simulink model "Lab6_jinjin"  (R2022a)
settings: Solver=VariableStepAuto  StartTime=0.0  StopTime=1200  RelTol=1e-3
libraries: matrix_library x4, sharedutil x2
settings Model: Creator=Administrator  LastModifiedBy=이진진
settings DebuggingCC: UnconnectedInputMsg=warning  UnconnectedOutputMsg=warning  UnconnectedLineMsg=warning
settings RTWCC: DLArmComputeVersion=19.05

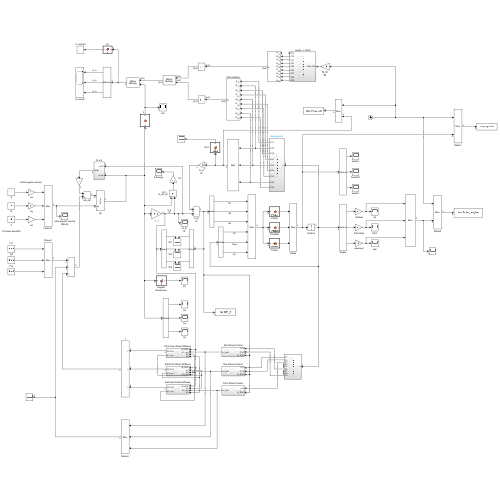
[thumbnail: Simulink's stored preview of the top-level diagram]
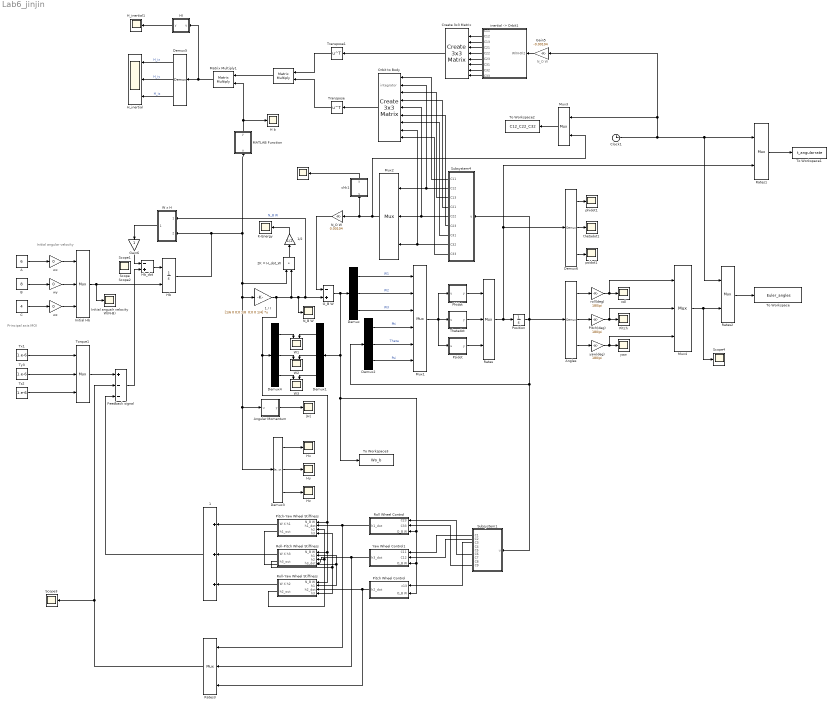
== system Lab6_jinjin ==
  note: Initial angular velocity
  note: Principal axis MOI
  note: N_O
      | W
  note: integrator
  " " : Scope
  "  " : Product  Multiplication=Matrix(*)
  " 1" : Sum  Inputs=+++
  1 / I : Gain  Gain="[1/6 0 0;0 1/8  0;0 0 1/4]"  Multiplication=Matrix(K*u)
  1/2 : Gain  Gain=1/2
  2K = H_dot_W : DotProduct  OutDataTypeStr=Inherit: Inherit via internal rule
  A : Constant  Value=6
  Angles : Demux  Outputs=3
      settings: DisplayOption=none
  Angular Momentum : MATLAB Function  TreatAsAtomicUnit=on
  B : Constant  Value=8
  C : Constant  Value=4
  Clock1 : Clock
  Create 3x3 Matrix : sharedutil/Create 3x3 Matrix  aMode=aMode
      settings: SourceProductBaseCode=AE,PW,DR,MT,VE
  Demux{,1..6} (7 alike) : Demux  Outputs=3
      settings: DisplayOption=none
  Feedback signal : Sum  Inputs=+--
  Gain5 : Gain  Gain=-0.00104
  Gain6 : Gain
  H b : Scope
  HI : MATLAB Function  TreatAsAtomicUnit=on
  H_inertial : Scope  NumInputPorts=3
  H_inertial1 : Scope
  Hb : Integrator  InitialConditionSource=external  InitialCondition=[0.2;0.3;0.4]
  Hb_dot : Sum  Inputs=-+
  Hx : Scope
  Hy : Scope
  Hz : Scope
  Initial Hb : Mux  Inputs=3
  Initial angualr velocity W(N-B) : Scope
  K-Energy : Scope
  MATLAB Function : MATLAB Function  TreatAsAtomicUnit=on
  Matrix Multiply1 : Product  Multiplication=Matrix(*)
  Mux1 : Mux  Inputs=6
  Mux2 : Mux  Inputs=3
  Mux3 : Mux  Inputs=2
  Mux4 : Mux  Inputs=3
  N_B W : Scope
  N_O W : Gain  Gain=0.00104
  O_B W : Sum  Inputs=-+
  Orbit to Body : sharedutil/Create 3x3 Matrix  aMode=aMode
      settings: SourceProductBaseCode=AE,PW,DR,MT,VE
  Phidot : MATLAB Function  TreatAsAtomicUnit=on
  Pitch : Scope
  Pitch Wheel Control : Subsystem
  Pitch(deg) : Gain  Gain=180/pi
  Pitch-Yaw Wheel Stiffness : Subsystem
  Position : Integrator  InitialCondition=[5*pi/180 5*pi/180 5*pi/180]
  Psidot : MATLAB Function  TreatAsAtomicUnit=on
  Rates : Mux  Inputs=3
  Rates1 : Mux  Inputs=2
  Rates2 : Mux  Inputs=2
  Rates3 : Mux  Inputs=3
  Roll Wheel Control : Subsystem
  Roll-Pitch Wheel Stiffness : Subsystem
  Roll-Yaw Wheel Stiffness : Subsystem
  Scope{,1..4} (5 alike) : Scope
  Subsystem1 : Subsystem
  Subsystem4 : Subsystem
  Thetadot : MATLAB Function  TreatAsAtomicUnit=on
  To Workspace : ToWorkspace  VariableName=Euler_angles  SampleTime=-1
  To Workspace1 : ToWorkspace  VariableName=t_angularrate  SaveFormat=Timeseries  SampleTime=-1
  To Workspace2 : ToWorkspace  VariableName=C12_C22_C32  SaveFormat=Timeseries  SampleTime=-1
  To Workspace3 : ToWorkspace  VariableName=Wo_b  SaveFormat=Timeseries  SampleTime=-1
  Torque1 : Mux  Inputs=3
  Transpose : Math  Operator=transpose
  Transpose1 : Math  Operator=transpose
  Tx1 : Constant  Value=1.e-6
  Ty3 : Constant  Value=1.e-6
  Tz2 : Constant  Value=1.e-6
  W x H : Subsystem
  W1 : Scope  NumInputPorts=2
  W2 : Scope  NumInputPorts=2
  W3 : Scope  NumInputPorts=2
  Yaw Wheel Control1 : Subsystem
  chk1 : MATLAB Function  TreatAsAtomicUnit=on
  "inertial -> Orbit1" : Subsystem
  phidot1 : Scope
  psidot1 : Scope
  roll : Scope
  roll(deg) : Gain  Gain=180/pi
  thetadot1 : Scope
  wx : Gain  Gain=0
  wy : Gain  Gain=0
  wz : Gain  Gain=0
  yaw : Scope
  yaw(deg) : Gain  Gain=180/pi
  |H| : Scope
  wires:
  Hb_dot/1 -> Hb/1
  W x H/1(WxH) -> Gain6/1
  Thetadot/1(y) -> Rates/2
  Demux2/1 -> Mux1/4  "Phi"
  Phidot/1(y) -> Rates/1
  Demux2/3 -> Mux1/6  "Psi"
  Demux1/2 -> W2/2
  Demux/3 -> Mux1/3  "W3"
  O_B W/1 -> Demux1/1, To Workspace3/1, Pitch Wheel Control/2(O_B W), Yaw Wheel Control1/3(O_B W), Roll Wheel Control/3(O_B W), Demux/1
  Subsystem4/2(C12) -> Mux2/1, Orbit to Body/2
  roll(deg)/1 -> Mux4/1, roll/1
  Angles/2 -> Pitch(deg)/1
  yaw(deg)/1 -> Mux4/3, yaw/1
  Angles/1 -> roll(deg)/1
  Demux/2 -> Mux1/2  "W2"
  "  "/1 -> Matrix Multiply1/1
  Subsystem4/1(C11) -> Orbit to Body/1
  Transpose/1 -> "  "/2
  Subsystem4/4(C21) -> Orbit to Body/4
  1 / I/1 -> Roll-Pitch Wheel Stiffness/1(N_B W), Roll-Yaw Wheel Stiffness/1(N_B W), Pitch-Yaw Wheel Stiffness/1(N_B W), Demux4/1, N_B W/1, W x H/1(in W), O_B W/2, 2K = H_dot_W/2  "N_B W"
  Transpose1/1 -> "  "/1
  Orbit to Body/1 -> Transpose/1
  Create 3x3 Matrix/1 -> Transpose1/1
  Demux1/3 -> W3/2
  Subsystem4/9(C33) -> Orbit to Body/9
  Angles/3 -> yaw(deg)/1
  2K = H_dot_W/1 -> 1/2/1
  chk1/1(y) -> " "/1
  Demux3/3 -> Hz/1
  Gain5/1 -> "inertial -> Orbit1"/1(W(N-O)2)
  Demux3/2 -> Hy/1
  Psidot/1(y) -> Rates/3
  Mux4/1 -> Scope4/1, Rates2/2
  Demux6/1 -> phidot1/1
  Demux6/2 -> thetadot1/1
  Subsystem4/6(C23) -> Orbit to Body/6
  Mux2/1 -> Mux3/2, chk1/1(u), N_O W/1
  Demux3/1 -> Hx/1
  Subsystem4/5(C22) -> Orbit to Body/5, Mux2/2
  N_O W/1 -> O_B W/1
  Demux/1 -> Mux1/1  "W1"
  Angular Momentum/1(y) -> |H|/1
  Demux2/2 -> Mux1/5  "Theta"
  Subsystem4/7(C31) -> Orbit to Body/7
  Hb/1 -> W x H/2(in Hb), Angular Momentum/1(u), Demux3/1, 1 / I/1, 2K = H_dot_W/1, MATLAB Function/1(u)
  Demux6/3 -> psidot1/1
  MATLAB Function/1(y) -> H b/1, Matrix Multiply1/2
  Mux1/1 -> Thetadot/1(u), Psidot/1(u), Phidot/1(u)
  Subsystem4/8(C32) -> Orbit to Body/8, Mux2/3
  Subsystem4/3(C13) -> Orbit to Body/3
  1/2/1 -> K-Energy/1
  C/1 -> wz/1
  B/1 -> wy/1
  Initial Hb/1 -> Hb/2, Initial angualr velocity W(N-B)/1
  wy/1 -> Initial Hb/2
  Ty3/1 -> Torque1/2
  wz/1 -> Initial Hb/3
  A/1 -> wx/1
  Torque1/1 -> Feedback signal/1
  Tz2/1 -> Torque1/3
  wx/1 -> Initial Hb/1
  Tx1/1 -> Torque1/1
  Feedback signal/1 -> Hb_dot/2
  Demux5/2 -> H_inertial/2  "H_iy"
  HI/1(y) -> H_inertial1/1
  Demux5/1 -> H_inertial/1  "H_ix"
  Matrix Multiply1/1 -> HI/1(u), Demux5/1
  Demux5/3 -> H_inertial/3  "H_iz"
  Position/1 -> Subsystem4/1(u), Subsystem1/1(u), Demux2/1, Angles/1
  Gain6/1 -> Hb_dot/1
  Rates1/1 -> To Workspace1/1
  Rates2/1 -> To Workspace/1
  Rates/1 -> Position/1, Rates1/2, Demux6/1
  Mux3/1 -> To Workspace2/1
  Clock1/1 -> Gain5/1, Mux3/1, Rates1/1, Rates2/1
  Subsystem1/3(C3) -> Pitch Wheel Control/1(c13)
  Subsystem1/1(C1) -> Yaw Wheel Control1/1(C11)
  Subsystem1/2(C2) -> Yaw Wheel Control1/2(C12)
  Subsystem1/6(C6) -> Roll Wheel Control/1(C23)
  Subsystem1/9(C9) -> Roll Wheel Control/2(C33)
  Roll Wheel Control/1(h1_dot) -> Rates3/1, Pitch-Yaw Wheel Stiffness/2(h1_dot)
  Pitch Wheel Control/1(h2_dot) -> Rates3/3, Roll-Yaw Wheel Stiffness/3(h2_dot)
  Yaw Wheel Control1/1(h3_dot) -> Rates3/2, Roll-Pitch Wheel Stiffness/4(h3_dot)
  Roll-Yaw Wheel Stiffness/2(h2_out) -> Pitch-Yaw Wheel Stiffness/3(h2), Roll-Pitch Wheel Stiffness/3(h2)
  Roll-Pitch Wheel Stiffness/2(h3_out) -> Roll-Yaw Wheel Stiffness/4(h3), Pitch-Yaw Wheel Stiffness/4(h3)
  Pitch-Yaw Wheel Stiffness/2(h1_out) -> Roll-Yaw Wheel Stiffness/2(h1), Roll-Pitch Wheel Stiffness/2(h1)
  Pitch-Yaw Wheel Stiffness/1(W X h1) -> " 1"/1
  Roll-Yaw Wheel Stiffness/1(W X h2) -> " 1"/3
  Roll-Pitch Wheel Stiffness/1(W X h3) -> " 1"/2
  " 1"/1 -> Feedback signal/3
  Rates3/1 -> Feedback signal/2, Scope3/1
  Demux1/1 -> W1/2
  Demux4/1 -> W1/1
  Demux4/2 -> W2/1
  Demux4/3 -> W3/1
  Pitch(deg)/1 -> Mux4/2, Pitch/1
  "inertial -> Orbit1"/9("C33 ") -> Create 3x3 Matrix/9
  "inertial -> Orbit1"/8("C32 ") -> Create 3x3 Matrix/8
  "inertial -> Orbit1"/5("C22 ") -> Create 3x3 Matrix/5
  "inertial -> Orbit1"/7("C31 ") -> Create 3x3 Matrix/7
  "inertial -> Orbit1"/6("C23 ") -> Create 3x3 Matrix/6
  "inertial -> Orbit1"/2("C12 ") -> Create 3x3 Matrix/2
  "inertial -> Orbit1"/3("C13 ") -> Create 3x3 Matrix/3
  "inertial -> Orbit1"/4("C21 ") -> Create 3x3 Matrix/4

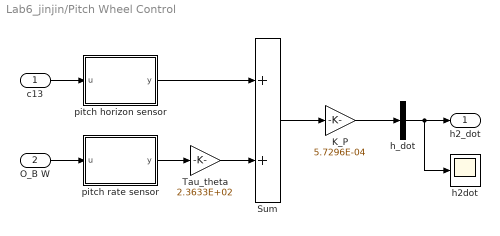
== system Lab6_jinjin/Pitch Wheel Control ==
  c13 : Inport
  O_B W : Inport  Port=2
  K_P : Gain  Gain=5.7296E-04
  Sum : Sum
  Tau_theta : Gain  Gain=2.3633E+02
  h2dot : Scope
  h_dot : Mux  Inputs=1
  pitch horizon sensor : MATLAB Function  TreatAsAtomicUnit=on
  pitch rate sensor : MATLAB Function  TreatAsAtomicUnit=on
  h2_dot : Outport
  wires:
  K_P/1 -> h_dot/1
  h_dot/1 -> h2dot/1, h2_dot/1
  pitch horizon sensor/1(y) -> Sum/1
  Tau_theta/1 -> Sum/2
  pitch rate sensor/1(y) -> Tau_theta/1
  O_B W/1 -> pitch rate sensor/1(u)
  c13/1 -> pitch horizon sensor/1(u)
  Sum/1 -> K_P/1

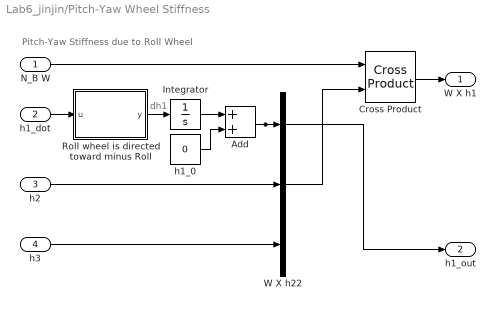
== system Lab6_jinjin/Pitch-Yaw Wheel Stiffness ==
  note: Pitch-Yaw Stiffness due to Roll Wheel
  note: dh1
  N_B W : Inport
  h1_dot : Inport  Port=2
  h2 : Inport  Port=3
  h3 : Inport  Port=4
  Add : Sum
  Cross Product : matrix_library/Cross Product
      settings: SourceProductBaseCode=SL
  Integrator : Integrator  InitialCondition=.0
  Roll wheel is directed toward minus Roll : MATLAB Function  TreatAsAtomicUnit=on
  W X h22 : Mux  Inputs=3
  h1_0 : Constant  Value=0  VectorParams1D=off
  W X h1 : Outport
  h1_out : Outport  Port=2
  wires:
  h1_dot/1 -> Roll wheel is directed toward minus Roll/1(u)
  Roll wheel is directed toward minus Roll/1(y) -> Integrator/1
  h1_0/1 -> Add/2
  Integrator/1 -> Add/1
  h3/1 -> W X h22/3
  N_B W/1 -> Cross Product/1
  W X h22/1 -> Cross Product/2
  Cross Product/1 -> W X h1/1
  h2/1 -> W X h22/2
  Add/1 -> h1_out/1, W X h22/1

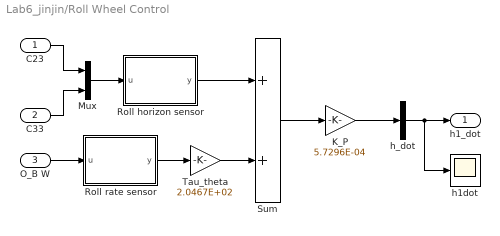
== system Lab6_jinjin/Roll Wheel Control ==
  C23 : Inport
  C33 : Inport  Port=2
  O_B W : Inport  Port=3
  K_P : Gain  Gain=5.7296E-04
  Mux : Mux  Inputs=2
  Roll horizon sensor : MATLAB Function  TreatAsAtomicUnit=on
  Roll rate sensor : MATLAB Function  TreatAsAtomicUnit=on
  Sum : Sum
  Tau_theta : Gain  Gain=2.0467E+02
  h1dot : Scope
  h_dot : Mux  Inputs=1
  h1_dot : Outport
  wires:
  K_P/1 -> h_dot/1
  h_dot/1 -> h1dot/1, h1_dot/1
  Roll horizon sensor/1(y) -> Sum/1
  Tau_theta/1 -> Sum/2
  Roll rate sensor/1(y) -> Tau_theta/1
  O_B W/1 -> Roll rate sensor/1(u)
  Sum/1 -> K_P/1
  C23/1 -> Mux/1
  C33/1 -> Mux/2
  Mux/1 -> Roll horizon sensor/1(u)

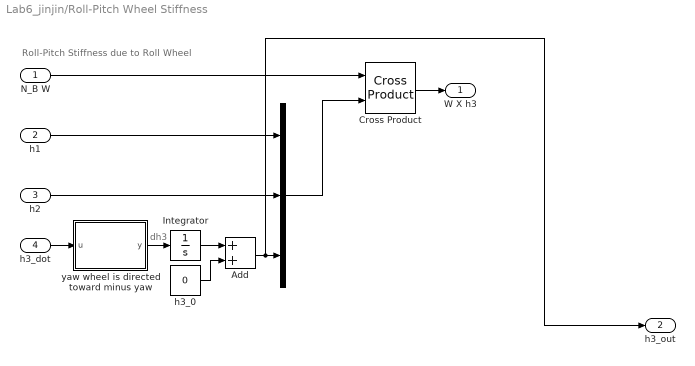
== system Lab6_jinjin/Roll-Pitch Wheel Stiffness ==
  note: Roll-Pitch Stiffness due to Roll Wheel
  note: dh3
  N_B W : Inport
  h1 : Inport  Port=2
  h2 : Inport  Port=3
  h3_dot : Inport  Port=4
  " " : Mux  Inputs=3
  Add : Sum
  Cross Product : matrix_library/Cross Product
      settings: SourceProductBaseCode=SL
  Integrator : Integrator  InitialCondition=.0
  h3_0 : Constant  Value=0  VectorParams1D=off
  yaw wheel is directed toward minus yaw : MATLAB Function  TreatAsAtomicUnit=on
  W X h3 : Outport
  h3_out : Outport  Port=2
  wires:
  h3_dot/1 -> yaw wheel is directed toward minus yaw/1(u)
  yaw wheel is directed toward minus yaw/1(y) -> Integrator/1
  h3_0/1 -> Add/2
  Integrator/1 -> Add/1
  N_B W/1 -> Cross Product/1
  " "/1 -> Cross Product/2
  Cross Product/1 -> W X h3/1
  Add/1 -> h3_out/1, " "/3
  h1/1 -> " "/1
  h2/1 -> " "/2

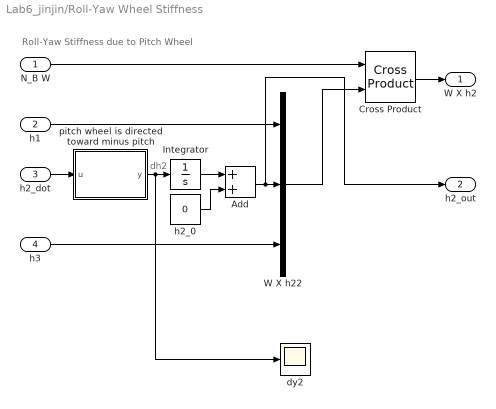
== system Lab6_jinjin/Roll-Yaw Wheel Stiffness ==
  note: Roll-Yaw Stiffness due to Pitch Wheel
  note: dh2
  N_B W : Inport
  h1 : Inport  Port=2
  h2_dot : Inport  Port=3
  h3 : Inport  Port=4
  Add : Sum
  Cross Product : matrix_library/Cross Product
      settings: SourceProductBaseCode=SL
  Integrator : Integrator  InitialCondition=.0
  W X h22 : Mux  Inputs=3
  dy2 : Scope
  h2_0 : Constant  Value=0  VectorParams1D=off
  pitch wheel is directed toward minus pitch : MATLAB Function  TreatAsAtomicUnit=on
  W X h2 : Outport
  h2_out : Outport  Port=2
  wires:
  h2_dot/1 -> pitch wheel is directed toward minus pitch/1(u)
  pitch wheel is directed toward minus pitch/1(y) -> dy2/1, Integrator/1
  Add/1 -> h2_out/1, W X h22/2
  h2_0/1 -> Add/2
  Integrator/1 -> Add/1
  h3/1 -> W X h22/3
  h1/1 -> W X h22/1
  N_B W/1 -> Cross Product/1
  W X h22/1 -> Cross Product/2
  Cross Product/1 -> W X h2/1

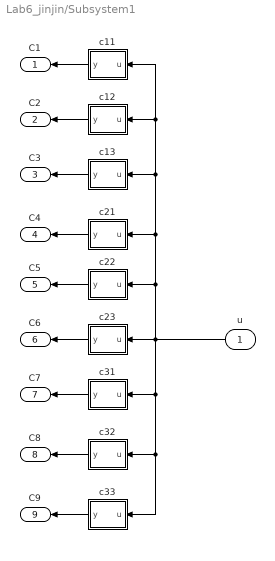
== system Lab6_jinjin/Subsystem1 ==
  u : Inport
  c11 : MATLAB Function  TreatAsAtomicUnit=on
  c12 : MATLAB Function  TreatAsAtomicUnit=on
  c13 : MATLAB Function  TreatAsAtomicUnit=on
  c21 : MATLAB Function  TreatAsAtomicUnit=on
  c22 : MATLAB Function  TreatAsAtomicUnit=on
  c23 : MATLAB Function  TreatAsAtomicUnit=on
  c31 : MATLAB Function  TreatAsAtomicUnit=on
  c32 : MATLAB Function  TreatAsAtomicUnit=on
  c33 : MATLAB Function  TreatAsAtomicUnit=on
  C1 : Outport
  C2 : Outport  Port=2
  C3 : Outport  Port=3
  C4 : Outport  Port=4
  C5 : Outport  Port=5
  C6 : Outport  Port=6
  C7 : Outport  Port=7
  C8 : Outport  Port=8
  C9 : Outport  Port=9
  wires:
  c32/1(y) -> C8/1
  c33/1(y) -> C9/1
  c23/1(y) -> C6/1
  c22/1(y) -> C5/1
  c12/1(y) -> C2/1
  c31/1(y) -> C7/1
  c13/1(y) -> C3/1
  c21/1(y) -> C4/1
  u/1 -> c32/1(u), c33/1(u), c31/1(u), c22/1(u), c13/1(u), c12/1(u), c11/1(u), c21/1(u), c23/1(u)
  c11/1(y) -> C1/1

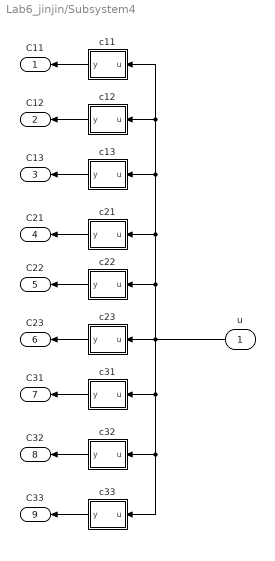
== system Lab6_jinjin/Subsystem4 ==
  u : Inport
  c11 : MATLAB Function  TreatAsAtomicUnit=on
  c12 : MATLAB Function  TreatAsAtomicUnit=on
  c13 : MATLAB Function  TreatAsAtomicUnit=on
  c21 : MATLAB Function  TreatAsAtomicUnit=on
  c22 : MATLAB Function  TreatAsAtomicUnit=on
  c23 : MATLAB Function  TreatAsAtomicUnit=on
  c31 : MATLAB Function  TreatAsAtomicUnit=on
  c32 : MATLAB Function  TreatAsAtomicUnit=on
  c33 : MATLAB Function  TreatAsAtomicUnit=on
  C11 : Outport
  C12 : Outport  Port=2
  C13 : Outport  Port=3
  C21 : Outport  Port=4
  C22 : Outport  Port=5
  C23 : Outport  Port=6
  C31 : Outport  Port=7
  C32 : Outport  Port=8
  C33 : Outport  Port=9
  wires:
  c22/1(y) -> C22/1
  c21/1(y) -> C21/1
  c23/1(y) -> C23/1
  c33/1(y) -> C33/1
  c32/1(y) -> C32/1
  c12/1(y) -> C12/1
  c11/1(y) -> C11/1
  u/1 -> c32/1(u), c33/1(u), c31/1(u), c22/1(u), c13/1(u), c12/1(u), c11/1(u), c21/1(u), c23/1(u)
  c31/1(y) -> C31/1
  c13/1(y) -> C13/1

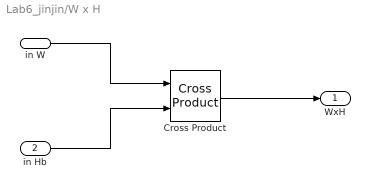
== system Lab6_jinjin/W x H ==
  in W : Inport
  in Hb : Inport  Port=2
  Cross Product : matrix_library/Cross Product
      settings: SourceProductBaseCode=SL
  WxH : Outport
  wires:
  in W/1 -> Cross Product/1
  Cross Product/1 -> WxH/1
  in Hb/1 -> Cross Product/2

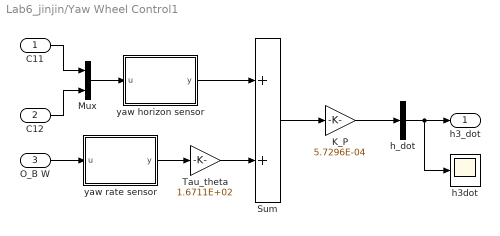
== system Lab6_jinjin/Yaw Wheel Control1 ==
  C11 : Inport
  C12 : Inport  Port=2
  O_B W : Inport  Port=3
  K_P : Gain  Gain=5.7296E-04
  Mux : Mux  Inputs=2
  Sum : Sum
  Tau_theta : Gain  Gain=1.6711E+02
  h3dot : Scope
  h_dot : Mux  Inputs=1
  yaw horizon sensor : MATLAB Function  TreatAsAtomicUnit=on
  yaw rate sensor : MATLAB Function  TreatAsAtomicUnit=on
  h3_dot : Outport
  wires:
  K_P/1 -> h_dot/1
  h_dot/1 -> h3dot/1, h3_dot/1
  yaw horizon sensor/1(y) -> Sum/1
  Tau_theta/1 -> Sum/2
  yaw rate sensor/1(y) -> Tau_theta/1
  O_B W/1 -> yaw rate sensor/1(u)
  Sum/1 -> K_P/1
  Mux/1 -> yaw horizon sensor/1(u)
  C11/1 -> Mux/1
  C12/1 -> Mux/2

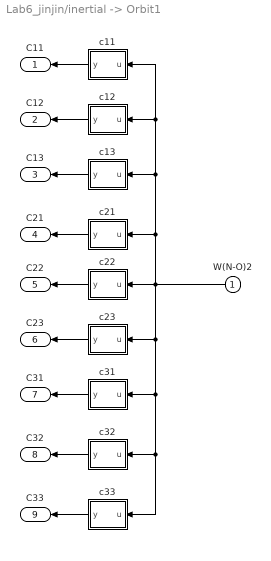
== system Lab6_jinjin/inertial -> Orbit1 ==
  W(N-O)2 : Inport
  c11 : MATLAB Function  TreatAsAtomicUnit=on
  c12 : MATLAB Function  TreatAsAtomicUnit=on
  c13 : MATLAB Function  TreatAsAtomicUnit=on
  c21 : MATLAB Function  TreatAsAtomicUnit=on
  c22 : MATLAB Function  TreatAsAtomicUnit=on
  c23 : MATLAB Function  TreatAsAtomicUnit=on
  c31 : MATLAB Function  TreatAsAtomicUnit=on
  c32 : MATLAB Function  TreatAsAtomicUnit=on
  c33 : MATLAB Function  TreatAsAtomicUnit=on
  "C11 " : Outport
  "C12 " : Outport  Port=2
  "C13 " : Outport  Port=3
  "C21 " : Outport  Port=4
  "C22 " : Outport  Port=5
  "C23 " : Outport  Port=6
  "C31 " : Outport  Port=7
  "C32 " : Outport  Port=8
  "C33 " : Outport  Port=9
  wires:
  c13/1(y) -> "C13 "/1
  c33/1(y) -> "C33 "/1
  c21/1(y) -> "C21 "/1
  c22/1(y) -> "C22 "/1
  c11/1(y) -> "C11 "/1
  c12/1(y) -> "C12 "/1
  W(N-O)2/1 -> c13/1(u), c12/1(u), c11/1(u), c21/1(u), c32/1(u), c33/1(u), c31/1(u), c23/1(u), c22/1(u)
  c32/1(y) -> "C32 "/1
  c31/1(y) -> "C31 "/1
  c23/1(y) -> "C23 "/1

== matlab function Lab6_jinjin/Angular Momentum ==
  data: u input; y output
function y = f(u)

y = sqrt(u(1)^2 + u(2)^2 + u(3)^2);

end

== matlab function Lab6_jinjin/Subsystem1/c12 ==
  data: u input; y output
function y = fcn(u)

y = sin(u(3))*cos(u(2));

== matlab function Lab6_jinjin/Subsystem1/c13 ==
  data: u input; y output
function y = fcn(u)

y = -sin(u(2));

== matlab function Lab6_jinjin/chk1 ==
  data: u input; y output
function y = chk1(u)

y = u(1)^2+u(2)^2+u(3)^2-1

end

== matlab function Lab6_jinjin/Subsystem4/c32 ==
  data: u input; y output
function y = fcn(u)

y = -cos(u(3))*sin(u(1))+sin(u(3))*sin(u(2))*cos(u(1));

== matlab function Lab6_jinjin/inertial -> Orbit1/c12 ==
  data: u input; y output
function y = fcn(u)

y = 0;

== matlab function Lab6_jinjin/Subsystem4/c33 ==
  data: u input; y output
function y = fcn(u)

y = cos(u(2))*cos(u(1));

== matlab function Lab6_jinjin/Subsystem1/c21 ==
  data: u input; y output
function y = fcn(u)

y = -sin(u(3))*cos(u(1))+cos(u(3))*sin(u(2))*sin(u(1));

== matlab function Lab6_jinjin/Subsystem1/c22 ==
  data: u input; y output
function y = fcn(u)

y = cos(u(3))*cos(u(1))+sin(u(3))*sin(u(2))*sin(u(1));

== matlab function Lab6_jinjin/Subsystem1/c23 ==
  data: u input; y output
function y = fcn(u)

y = cos(u(2))*sin(u(1));

== matlab function Lab6_jinjin/Subsystem1/c31 ==
  data: u input; y output
function y = fcn(u)

y = sin(u(3))*sin(u(1))+cos(u(3))*sin(u(2))*cos(u(1));

== matlab function Lab6_jinjin/Subsystem1/c32 ==
  data: u input; y output
function y = fcn(u)

y = -cos(u(3))*sin(u(1))+sin(u(3))*sin(u(2))*cos(u(1));

== matlab function Lab6_jinjin/Subsystem1/c33 ==
  data: u input; y output
function y = fcn(u)

y = cos(u(2))*cos(u(1));

== matlab function Lab6_jinjin/Pitch Wheel Control/pitch horizon sensor ==
  data: u input; y output
function y = fcn(u)

y = -u(1);

== matlab function Lab6_jinjin/MATLAB Function ==
  data: u input; y output
function y = f(u)

y = zeros(3,1);

y(1,1) = u(1);
y(2,1) = u(2);
y(3,1) = u(3);

== matlab function Lab6_jinjin/Pitch Wheel Control/pitch rate sensor ==
  data: u input; y output
function y = fcn(u)

y = u(2);

== matlab function Lab6_jinjin/inertial -> Orbit1/c13 ==
  data: u input; y output
function y = fcn(u)

y = -sin(u);

== matlab function Lab6_jinjin/Roll Wheel Control/Roll horizon sensor ==
  data: u input; y output
function y = fcn(u)

y = atan(u(1)/u(2));

== matlab function Lab6_jinjin/HI ==
  data: u input; y output
function y = fcn(u)

y = sqrt((u(1)^2+u(2)^2+u(3)^2));

== matlab function Lab6_jinjin/Roll Wheel Control/Roll rate sensor ==
  data: u input; y output
function y = fcn(u)

y = u(1);

== matlab function Lab6_jinjin/Yaw Wheel Control1/yaw horizon sensor ==
  data: u input; y output
function y = fcn(u)

y = atan(u(2)/u(1));

== matlab function Lab6_jinjin/Yaw Wheel Control1/yaw rate sensor ==
  data: u input; y output
function y = fcn(u)

y = u(3);

== matlab function Lab6_jinjin/Pitch-Yaw Wheel Stiffness/Roll wheel is directed toward minus Roll ==
  data: u input; y output
function y = fcn(u)

y = -u(1);

== matlab function Lab6_jinjin/Roll-Pitch Wheel Stiffness/yaw wheel is directed toward minus yaw ==
  data: u input; y output
function y = fcn(u)

y = -u(1);

== matlab function Lab6_jinjin/Roll-Yaw Wheel Stiffness/pitch wheel is directed toward minus pitch ==
  data: u input; y output
function y = fcn(u)

y = -u(1);

== matlab function Lab6_jinjin/inertial -> Orbit1/c21 ==
  data: u input; y output
function y = fcn(u)

y = 0;

== matlab function Lab6_jinjin/inertial -> Orbit1/c22 ==
  data: u input; y output
function y = fcn(u)

y = 1;

== matlab function Lab6_jinjin/Phidot ==
  data: u input; y output
function y = Phidot(u)

y = u(1) + sin(u(4))*tan(u(5))*u(2) + cos(u(4))*tan(u(5))*u(3);

end

== matlab function Lab6_jinjin/inertial -> Orbit1/c23 ==
  data: u input; y output
function y = fcn(u)

y = 0;

== matlab function Lab6_jinjin/inertial -> Orbit1/c31 ==
  data: u input; y output
function y = fcn(u)

y = sin(u);

== matlab function Lab6_jinjin/inertial -> Orbit1/c32 ==
  data: u input; y output
function y = fcn(u)

y = 0;

== matlab function Lab6_jinjin/inertial -> Orbit1/c33 ==
  data: u input; y output
function y = fcn(u)

y = cos(u);

== matlab function Lab6_jinjin/Psidot ==
  data: u input; y output
function y = Psidot(u)

y = (sin(u(4))/cos(u(5)))*u(2) + (cos(u(4))/cos(u(5))*u(3));

end

== matlab function Lab6_jinjin/Subsystem4/c12 ==
  data: u input; y output
function y = fcn(u)

y = sin(u(3))*cos(u(2));

== matlab function Lab6_jinjin/Subsystem4/c13 ==
  data: u input; y output
function y = fcn(u)

y = -sin(u(2));

== matlab function Lab6_jinjin/Subsystem4/c21 ==
  data: u input; y output
function y = fcn(u)

y = -sin(u(3))*cos(u(1))+cos(u(3))*sin(u(2))*sin(u(1));

== matlab function Lab6_jinjin/Subsystem4/c22 ==
  data: u input; y output
function y = fcn(u)

y = cos(u(3))*cos(u(1))+sin(u(3))*sin(u(2))*sin(u(1));

== matlab function Lab6_jinjin/inertial -> Orbit1/c11 ==
  data: u input; y output
function y = fcn(u)

y = cos(u);

== matlab function Lab6_jinjin/Subsystem4/c23 ==
  data: u input; y output
function y = fcn(u)

y = cos(u(2))*sin(u(1));

== matlab function Lab6_jinjin/Subsystem4/c31 ==
  data: u input; y output
function y = fcn(u)

y = sin(u(3))*sin(u(1))+cos(u(3))*sin(u(2))*cos(u(1));

== matlab function Lab6_jinjin/Subsystem4/c11 ==
  data: u input; y output
function y = fcn(u)

y = cos(u(3))*cos(u(2));

== matlab function Lab6_jinjin/Thetadot ==
  data: u input; y output
function y = Thetadot(u)

y = cos(u(4))*u(2) - sin(u(4))*u(3);

end

== matlab function Lab6_jinjin/Subsystem1/c11 ==
  data: u input; y output
function y = fcn(u)

y = cos(u(3))*cos(u(2));
